simulink model "FiveStateABSforMotorcycle"  (R2025b)
settings: configuration reference "VehicleFixed1ms" (kept outside this file)
undefined symbols (not defined in the file): DiscIntNeverNeededParam
libraries: simulink x3, autolibutils x1
settings Model: DataDictionary=VirtualMotoTemplate.sldd  ModifiedByFormat=The MathWorks, Inc.  Creator=The MathWorks, Inc.  LastModifiedBy=The MathWorks, Inc.
settings ConfigSetRef: SourceName=VehicleFixed1ms

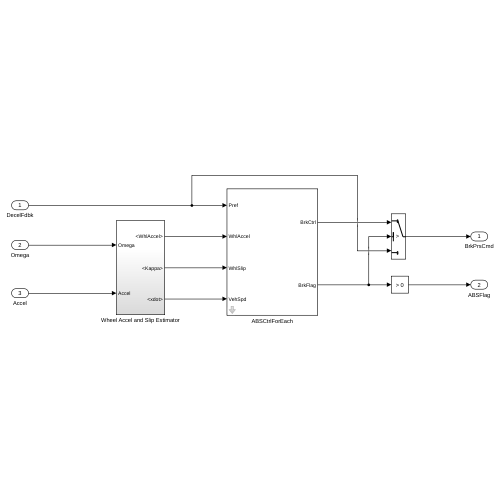
[thumbnail: Simulink's stored preview of the top-level diagram]
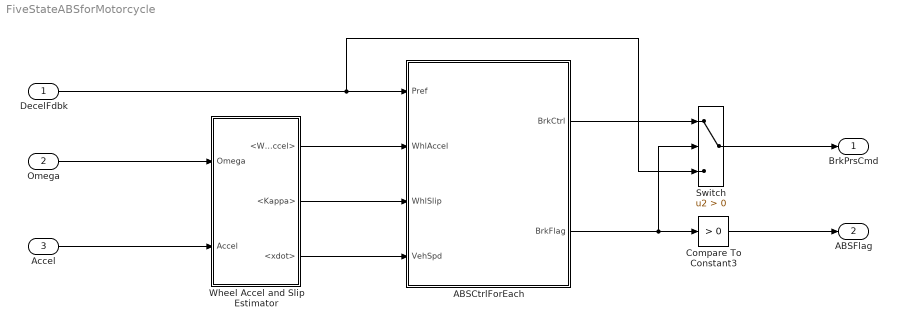
== system FiveStateABSforMotorcycle ==
  DecelFdbk : Inport  PortDimensions=2
  Omega : Inport  Port=2  PortDimensions=2
  Accel : Inport  Port=3  PortDimensions=3
  ABSCtrlForEach : Subsystem  mask(Five-State ABS Control){Re=0.31, KappaOpt=[0, -0.1], WhlAccelOpt=[-5, -5], v1=[-55, -55], v5=[10, 10], v4=[30, 30], a2=[5, 5], b=[0, 0], A=[5, 5], a1=[4, 4], aMode=2}
      mask prompts: Re "Wheel effective radius, Re [m]:"; KappaOpt "Desired wheel slip ratio, KappaOpt [-]:"; WhlAccelOpt "Desired wheel acceleration, WhlAccelOpt [m/s^2]:"; v1 "Braking pressure declining rate, v1 [-]:"; v5 "Secondary braking pressure rising rate, v5 [-]:"; v4 "Braking pressure rising rate, v4 [-]:"; a2 "Threshold of State 1, a2 [m/s^2]:"; b "Threshold of State 2, b [m/s^2]:"; A "Threshold of State 3 and 4, A [m/s^2]:"; a1 "Threshold of State 5, a1 [m/s^2]:"
      mask help: This block determines brake pressure varying rate for each wheel once the ABS controller is activated. During ABS control, only wheel speed is directly regulated.
      mask init:
      | [~]=vehdynicon('vehdynblk',gcb);
      mask DialogControl vehParamGroup Prompt: Vehicle Parameter
      mask DialogControl ParameterGroupVar Prompt: Desired Control Parameters
      mask DialogControl Container3 Prompt: Braking Pressure Rates
      mask DialogControl Container4 Prompt: Wheel Acceleration Thresholds
  Compare To Constant3 : simulink/Logic and Bit Operations/Compare To Constant  relop=>  const=0  OutDataTypeStr=boolean  ZeroCross=off
  Switch : Switch  Criteria=u2 > Threshold  SaturateOnIntegerOverflow=off  InputSameDT=off
  Wheel Accel and Slip Estimator : Subsystem
  BrkPrsCmd : Outport
  ABSFlag : Outport  Port=2  OutDataTypeStr=boolean  PortDimensions=2
  wires:
  Accel/1 -> Wheel Accel and Slip Estimator/2(Accel)
  Wheel Accel and Slip Estimator/1(<WhlAccel>) -> ABSCtrlForEach/2(WhlAccel)
  ABSCtrlForEach/1(BrkCtrl) -> Switch/1
  Omega/1 -> Wheel Accel and Slip Estimator/1(Omega)
  Wheel Accel and Slip Estimator/2(<Kappa>) -> ABSCtrlForEach/3(WhlSlip)
  DecelFdbk/1 -> Switch/3, ABSCtrlForEach/1(Pref)
  Switch/1 -> BrkPrsCmd/1
  Wheel Accel and Slip Estimator/3(<xdot>) -> ABSCtrlForEach/4(VehSpd)
  ABSCtrlForEach/2(BrkFlag) -> Compare To Constant3/1, Switch/2
  Compare To Constant3/1 -> ABSFlag/1

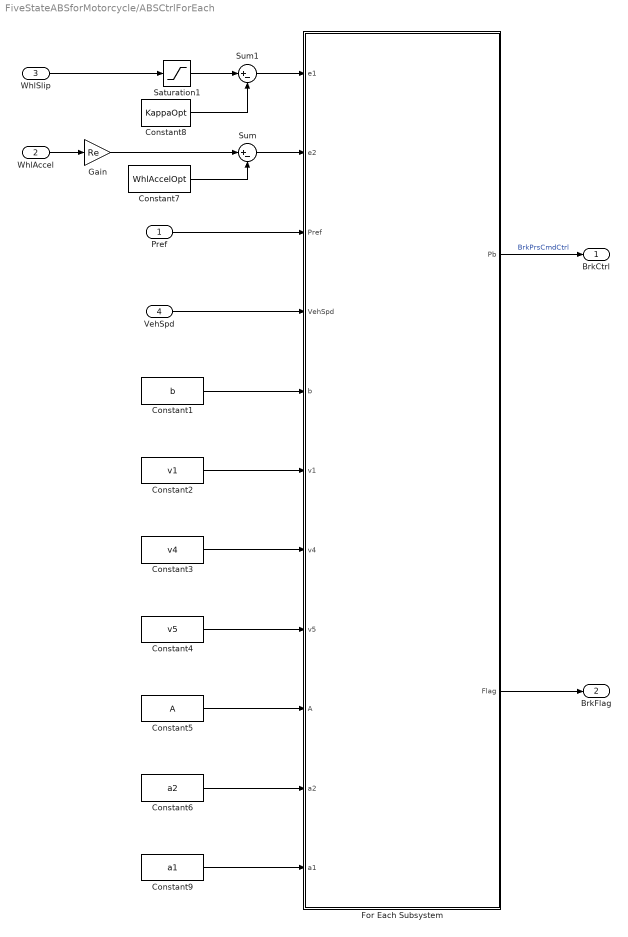
== system FiveStateABSforMotorcycle/ABSCtrlForEach ==
  Pref : Inport
  WhlAccel : Inport  Port=2
  WhlSlip : Inport  Port=3
  VehSpd : Inport  Port=4
  Constant1 : Constant  Value=b
  Constant2 : Constant  Value=v1
  Constant3 : Constant  Value=v4
  Constant4 : Constant  Value=v5
  Constant5 : Constant  Value=A
  Constant6 : Constant  Value=a2
  Constant7 : Constant  Value=WhlAccelOpt
  Constant8 : Constant  Value=KappaOpt
  Constant9 : Constant  Value=a1
  For Each Subsystem : Subsystem  TreatAsAtomicUnit=on
  Gain : Gain  Gain=Re
  Saturation1 : Saturate  UpperLimit=1  LowerLimit=-1
  Sum : Sum  Inputs=|+-
  Sum1 : Sum  Inputs=|+-
  BrkCtrl : Outport
  BrkFlag : Outport  Port=2
  wires:
  Constant9/1 -> For Each Subsystem/11(a1)
  Constant6/1 -> For Each Subsystem/10(a2)
  Constant5/1 -> For Each Subsystem/9(A)
  Constant4/1 -> For Each Subsystem/8(v5)
  Constant3/1 -> For Each Subsystem/7(v4)
  Constant2/1 -> For Each Subsystem/6(v1)
  Constant1/1 -> For Each Subsystem/5(b)
  Sum/1 -> For Each Subsystem/2(e2)
  Pref/1 -> For Each Subsystem/3(Pref)
  For Each Subsystem/1(Pb) -> BrkCtrl/1  "BrkPrsCmdCtrl"
  VehSpd/1 -> For Each Subsystem/4(VehSpd)
  For Each Subsystem/2(Flag) -> BrkFlag/1
  Saturation1/1 -> Sum1/1
  WhlAccel/1 -> Gain/1
  Sum1/1 -> For Each Subsystem/1(e1)
  Constant7/1 -> Sum/2
  WhlSlip/1 -> Saturation1/1
  Constant8/1 -> Sum1/2
  Gain/1 -> Sum/1

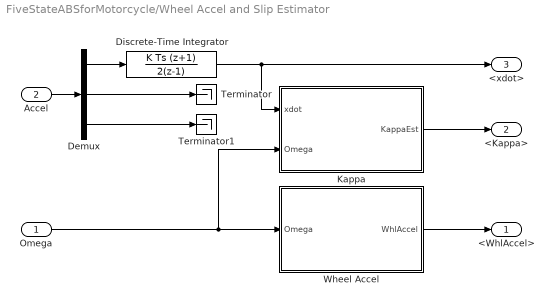
== system FiveStateABSforMotorcycle/Wheel Accel and Slip Estimator ==
  Omega : Inport
  Accel : Inport  Port=2
  Demux : Demux  Outputs=3
  Discrete-Time Integrator : DiscreteIntegrator  IntegratorMethod=Integration: Trapezoidal  SampleTime=-1  LimitOutput=on  LowerSaturationLimit=0  ICPrevOutput=DiscIntNeverNeededParam  ICPrevScaledInput=DiscIntNeverNeededParam
  Kappa : Subsystem  TreatAsAtomicUnit=on
  Terminator : Terminator
  Terminator1 : Terminator
  Wheel Accel : Subsystem  TreatAsAtomicUnit=on
  <WhlAccel> : Outport
  <Kappa> : Outport  Port=2
  <xdot> : Outport  Port=3
  wires:
  Demux/1 -> Discrete-Time Integrator/1
  Wheel Accel/1(WhlAccel) -> <WhlAccel>/1
  Kappa/1(KappaEst) -> <Kappa>/1
  Omega/1 -> Kappa/2(Omega), Wheel Accel/1(Omega)
  Demux/3 -> Terminator1/1
  Demux/2 -> Terminator/1
  Discrete-Time Integrator/1 -> <xdot>/1, Kappa/1(xdot)
  Accel/1 -> Demux/1

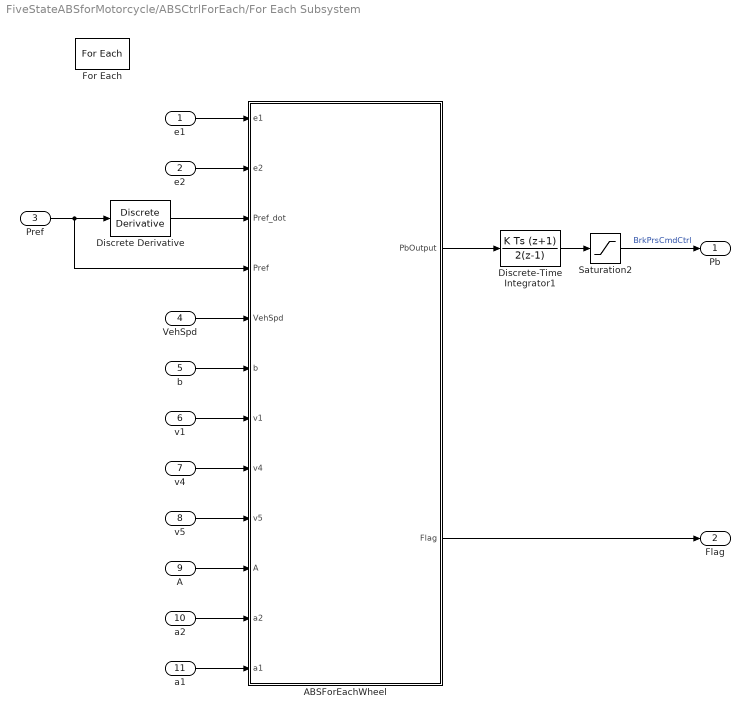
== system FiveStateABSforMotorcycle/ABSCtrlForEach/For Each Subsystem ==
  e1 : Inport  Partition=on  PartitionDimension=1  PartitionWidth=1  PartitionOffset=0
  e2 : Inport  Port=2  Partition=on  PartitionDimension=1  PartitionWidth=1  PartitionOffset=0
  Pref : Inport  Port=3  Partition=on  PartitionDimension=1  PartitionWidth=1  PartitionOffset=0
  VehSpd : Inport  Port=4
  b : Inport  Port=5  Partition=on  PartitionDimension=1  PartitionWidth=1  PartitionOffset=0
  v1 : Inport  Port=6  Partition=on  PartitionDimension=1  PartitionWidth=1  PartitionOffset=0
  v4 : Inport  Port=7  Partition=on  PartitionDimension=1  PartitionWidth=1  PartitionOffset=0
  v5 : Inport  Port=8  Partition=on  PartitionDimension=1  PartitionWidth=1  PartitionOffset=0
  A : Inport  Port=9  Partition=on  PartitionDimension=1  PartitionWidth=1  PartitionOffset=0
  a2 : Inport  Port=10  Partition=on  PartitionDimension=1  PartitionWidth=1  PartitionOffset=0
  a1 : Inport  Port=11  Partition=on  PartitionDimension=1  PartitionWidth=1  PartitionOffset=0
  ABSForEachWheel : Stateflow chart  InitFcn=[~]=vehdynicon('vehdynblk',gcb);  TreatAsAtomicUnit=on
  Discrete Derivative : simulink/Discrete/Discrete Derivative  gainval=1.0  ICPrevScaledInput=0.0  OutMin=[]  OutMax=[]  OutDataType=fixdt(1, 16)  OutScaling=2^-10  DoSatur=off
  Discrete-Time Integrator1 : DiscreteIntegrator  IntegratorMethod=Integration: Trapezoidal  SampleTime=-1  ICPrevOutput=DiscIntNeverNeededParam  ICPrevScaledInput=DiscIntNeverNeededParam
  For Each : ForEach  DisableCoverage=on
  Saturation2 : Saturate  UpperLimit=1  LowerLimit=0
  Pb : Outport  ConcatenationDimension=1
  Flag : Outport  Port=2  ConcatenationDimension=1
  wires:
  a1/1 -> ABSForEachWheel/12(a1)
  a2/1 -> ABSForEachWheel/11(a2)
  A/1 -> ABSForEachWheel/10(A)
  v5/1 -> ABSForEachWheel/9(v5)
  v4/1 -> ABSForEachWheel/8(v4)
  v1/1 -> ABSForEachWheel/7(v1)
  b/1 -> ABSForEachWheel/6(b)
  Discrete Derivative/1 -> ABSForEachWheel/3(Pref_dot)
  ABSForEachWheel/1(PbOutput) -> Discrete-Time Integrator1/1
  Discrete-Time Integrator1/1 -> Saturation2/1
  Pref/1 -> ABSForEachWheel/4(Pref), Discrete Derivative/1
  ABSForEachWheel/2(Flag) -> Flag/1
  Saturation2/1 -> Pb/1  "BrkPrsCmdCtrl"
  VehSpd/1 -> ABSForEachWheel/5(VehSpd)
  e2/1 -> ABSForEachWheel/2(e2)
  e1/1 -> ABSForEachWheel/1(e1)

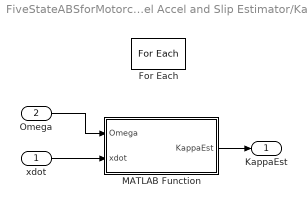
== system FiveStateABSforMotorcycle/Wheel Accel and Slip Estimator/Kappa ==
  xdot : Inport
  Omega : Inport  Port=2  PortDimensions=1  Partition=on  PartitionDimension=1  PartitionWidth=1  PartitionOffset=0
  For Each : ForEach  DisableCoverage=on
  MATLAB Function : MATLAB Function  TreatAsAtomicUnit=on
  KappaEst : Outport  ConcatenationDimension=1
  wires:
  Omega/1 -> MATLAB Function/1(Omega)
  xdot/1 -> MATLAB Function/2(xdot)
  MATLAB Function/1(KappaEst) -> KappaEst/1

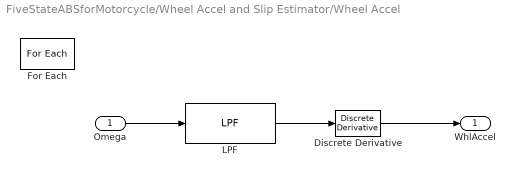
== system FiveStateABSforMotorcycle/Wheel Accel and Slip Estimator/Wheel Accel ==
  Omega : Inport  PortDimensions=1  Partition=on  PartitionDimension=1  PartitionWidth=1  PartitionOffset=0
  Discrete Derivative : simulink/Discrete/Discrete Derivative  gainval=1.0  ICPrevScaledInput=0.0  OutMin=[]  OutMax=[]  OutDataType=fixdt(1, 16)  OutScaling=2^-10  DoSatur=off
  For Each : ForEach  DisableCoverage=on
  LPF : autolibutils/LPF  w=5  aMode=2
  WhlAccel : Outport  ConcatenationDimension=1
  wires:
  Discrete Derivative/1 -> WhlAccel/1
  LPF/1 -> Discrete Derivative/1
  Omega/1 -> LPF/1

== stateflow chart FiveStateABSforMotorcycle/ABSCtrlForEach/For Each Subsystem/ABSForEachWheel ==
  state ABSOff
    entry:
    PbOutput = Pref_dot;
    Flag = 0;
    during:
    PbOutput = Pref_dot;
  state Normal
    entry:
    PbOutput = Pref_dot;
    Flag = 0;
    during:
    PbOutput = Pref_dot;
  state ABSOn
    state Phase1
      entry:
      PbOutput = v1;
      Flag = 1;
    state Phase5
      entry:
      PbOutput = v5;
      Flag = 5;
    state Phase2
      entry:
      PbOutput = 0;
      Flag = 2;
    state Phase4
      entry:
      PbOutput = 0;
      Flag = 4;
    state Phase3
      entry:
      PbOutput = v4;
      Flag = 3;
    (default) -> Phase1
    Phase5 -> Phase1 : [e2 < a2]
    Phase1 -> Phase2 : [e2 >= b]
    Phase4 -> Phase5 : [e2 <= a1]
    Phase2 -> Phase3 : [e2 >= A]
    Phase3 -> Phase4 : [e2 < A]
  (default) -> ABSOff
  ABSOn -> ABSOff : [abs(VehSpd) < 0.5 || Pref <= 0]
  Normal -> ABSOff [order 2] : [Pref <= 0]
  ABSOff -> Normal : [Pref > 0.1 && e2 < a2]
  Normal -> ABSOn [order 1] : [e1 < 0]
  data: e1 input; e2 input; PbOutput output; Flag output; Pref_dot input; Pref input; VehSpd input; b input; v1 input; v4 input; v5 input; A input; a2 input; a1 input

== matlab function FiveStateABSforMotorcycle/Wheel Accel and Slip Estimator/Kappa/MATLAB Function ==
  data: Omega input; xdot input; KappaEst output
function KappaEst = fcn(Omega, xdot)

Re = 0.29;
KappaEst = 0;
WhlSpd = Omega * Re;

if xdot*WhlSpd ~= 0
    KappaEst = (WhlSpd - xdot)/max([abs(xdot) abs(WhlSpd)]);
end
